simulink model "on_off_lampara_stt"  (R2018a)
settings: Solver=VariableStepAuto  StartTime=0.0  StopTime=inf  RelTol=1e-3
settings Model: Creator=carma  LastModifiedBy=carma

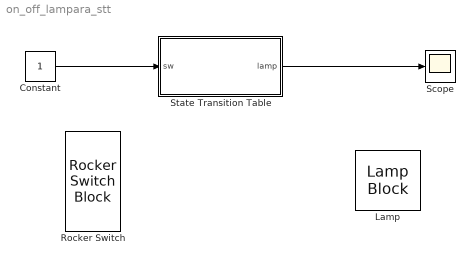
== system on_off_lampara_stt ==
  Constant : Constant
  Lamp : LampBlock  WebBlockId=5
  Rocker Switch : RockerSwitchBlock  WebBlockId=4
      settings: Values={{'Off', 'On'}, [0 1]}
  Scope : Scope
  State Transition Table : State Transition Table  TreatAsAtomicUnit=on
  wires:
  Constant/1 -> State Transition Table/1(sw)
  State Transition Table/1(lamp) -> Scope/1

== stateflow chart on_off_lampara_stt/State Transition Table ==
  state OFF
    entry:
    lamp=0;
  state ON
    entry:
    lamp=1;
  (default) -> OFF
  OFF -> (junction 19) [order 2]
  (junction 19) -> OFF
  OFF -> ON [order 1] : [sw==1]
  ON -> OFF [order 1] : [sw==0]
  ON -> (junction 23) [order 2]
  (junction 23) -> ON
  data: sw input; lamp output
